simulink model "SimplePendulumMotion"  (R2022b)
settings: Solver=ode23tb  StartTime=0.0  StopTime=10.0  MaxStep=.0001  RelTol=1e-3
values from neighbouring files (symbols this model uses):
  b = .5    (= 0.5)    [SimplePendulumMotion_Parameters.m]
  g = 9.81    [SimplePendulumMotion_Parameters.m]
  L = lengthValues(i)    [SimplePendulumMotion_Parameters.m]
settings Model: Creator=MOHAMED  LastModifiedBy=MOHAMED

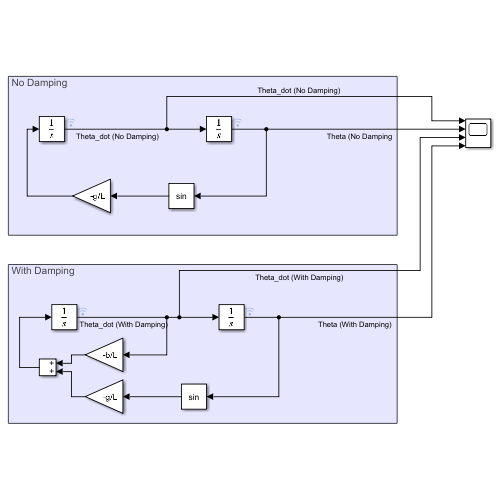
[thumbnail: Simulink's stored preview of the top-level diagram]
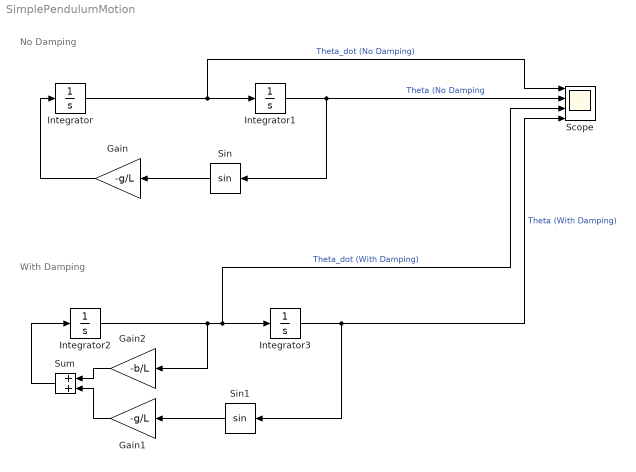
== system SimplePendulumMotion ==
  note: No Damping
  note: With Damping
  Gain : Gain  Gain=-g/L
  Gain1 : Gain  Gain=-g/L
  Gain2 : Gain  Gain=-b/L
  Integrator : Integrator
  Integrator1 : Integrator  InitialCondition=pi/4
  Integrator2 : Integrator
  Integrator3 : Integrator  InitialCondition=pi/4
  Scope : Scope  NumInputPorts=4
  Sin : Trigonometry
  Sin1 : Trigonometry
  Sum : Sum
  wires:
  Integrator/1 -> Scope/1, Integrator1/1  "Theta_dot (No Damping)"
  Sin/1 -> Gain/1
  Integrator1/1 -> Sin/1, Scope/2  "Theta (No Damping"
  Gain/1 -> Integrator/1
  Integrator2/1 -> Gain2/1, Scope/3, Integrator3/1  "Theta_dot (With Damping)"
  Sin1/1 -> Gain1/1
  Integrator3/1 -> Sin1/1, Scope/4  "Theta (With Damping)"
  Gain2/1 -> Sum/1
  Gain1/1 -> Sum/2
  Sum/1 -> Integrator2/1
